simulink model "elevator"  (R2020a)
settings: Solver=VariableStepAuto  StartTime=0.0  StopTime=inf  RelTol=1e-3
PreLoadFcn:
  | slplc.api.loadDataTypes;
undefined symbols (not defined in the file): BOOL, DINT, INT, slplc
libraries: simulink x1
(part 23 of 38)

== system elevator/PLCControllerSuite/__Logic/Task/Program/__Logic/XIO2/BlockEnableRead ==
  __CoreLabelRead : Subsystem  Tag=CoreVarReadBlock  DisableCoverage=on  TreatAsAtomicUnit=on  mask{PLCBlockType=CoreLabelRead}
      mask init:
      | slplc.callbacks.initRoutineLabelRead(gcb);
      mask Help: web([docroot '/plccoder/ref/__corelabelread' '.html']);
      mask DialogControl PLCBlockTitle Prompt: Core Label Read
  Out1 : Outport  VectorParamsAs1DForOutWhenUnconnected=off
  wires:
  __CoreLabelRead/1(Out1) -> Out1/1

== system elevator/PLCControllerSuite/__Logic/Task/Program/__Logic/XIO2/Instruction_Enable ==
  Rung-condition-in : Inport  OutDataTypeStr=BOOL
  Enable : EnablePort
  Logical Operator : Logic  OutDataTypeStr=BOOL
  NOT : Logic  DisableCoverage=on  Operator=NOT  IconShape=distinctive  OutDataTypeStr=BOOL
  __CoreVarRead : Subsystem  Tag=CoreVarReadBlock  DisableCoverage=on  TreatAsAtomicUnit=on  mask{PLCBlockType=CoreVarRead}
      mask init:
      | slplc.callbacks.initCoreVariable(gcb, 'read');
      mask Help: web([docroot '/plccoder/ref/__corevarread' '.html']);
      mask DialogControl PLCBlockTitle Prompt: Core Variable Read
  Rung-condition-out : Outport  VectorParamsAs1DForOutWhenUnconnected=off
  wires:
  NOT/1 -> Logical Operator/2  "~DataBit"
  __CoreVarRead/1(y) -> NOT/1  "DataBit"
  Logical Operator/1 -> Rung-condition-out/1  "Rung-condition-out"
  Rung-condition-in/1 -> Logical Operator/1  "Rung-condition-in"

== system elevator/PLCControllerSuite/__Logic/Task/Program/__Logic/XIO2/RungInOverride ==
  In1 : Inport
  AND : Logic  AllPortsSameDT=off  OutDataTypeStr=boolean
  ForceRungInFalseRead : Subsystem  DisableCoverage=on  TreatAsAtomicUnit=on  mask{PLCLabelTag=_Force_RungIn_False, PLCBlockType=ForceRungInFalseRead}
      mask prompts: PLCLabelTag "Label Tag:"
      mask init:
      | block = gcb;
      | maskObj = Simulink.Mask.get(block);
      | maskObj.Display = sprintf('disp(''%s'');', PLCLabelTag);
      mask Help: web([docroot '/plccoder/ref/forcerunginfalseread' '.html']);
      mask DialogControl PLCBlockTitle Prompt: Force Rung-In False Read
      mask Display: disp('_Force_RungIn_False');
  NOT : Logic  Operator=NOT  IconShape=distinctive  AllPortsSameDT=off  OutDataTypeStr=boolean
  Out1 : Outport  VectorParamsAs1DForOutWhenUnconnected=off
  wires:
  NOT/1 -> AND/1
  ForceRungInFalseRead/1(Out1) -> NOT/1
  In1/1 -> AND/2
  AND/1 -> Out1/1

== system elevator/PLCControllerSuite/__Logic/Task/Program/__Logic/XIO2/__CoreVarRead ==
  DataRead : DataStoreRead  DataStoreName=xxx_PLC_VAR_AtFloor2
  y : Outport  VectorParamsAs1DForOutWhenUnconnected=off
  wires:
  DataRead/1 -> y/1

== system elevator/PLCControllerSuite/__Logic/Task/Program/__Logic/XIO20/BlockEnableRead ==
  __CoreLabelRead : Subsystem  Tag=CoreVarReadBlock  DisableCoverage=on  TreatAsAtomicUnit=on  mask{PLCBlockType=CoreLabelRead}
      mask init:
      | slplc.callbacks.initRoutineLabelRead(gcb);
      mask Help: web([docroot '/plccoder/ref/__corelabelread' '.html']);
      mask DialogControl PLCBlockTitle Prompt: Core Label Read
  Out1 : Outport  VectorParamsAs1DForOutWhenUnconnected=off
  wires:
  __CoreLabelRead/1(Out1) -> Out1/1

== system elevator/PLCControllerSuite/__Logic/Task/Program/__Logic/XIO20/Instruction_Enable ==
  Rung-condition-in : Inport  OutDataTypeStr=BOOL
  Enable : EnablePort
  Logical Operator : Logic  OutDataTypeStr=BOOL
  NOT : Logic  DisableCoverage=on  Operator=NOT  IconShape=distinctive  OutDataTypeStr=BOOL
  __CoreVarRead : Subsystem  Tag=CoreVarReadBlock  DisableCoverage=on  TreatAsAtomicUnit=on  mask{PLCBlockType=CoreVarRead}
      mask init:
      | slplc.callbacks.initCoreVariable(gcb, 'read');
      mask Help: web([docroot '/plccoder/ref/__corevarread' '.html']);
      mask DialogControl PLCBlockTitle Prompt: Core Variable Read
  Rung-condition-out : Outport  VectorParamsAs1DForOutWhenUnconnected=off
  wires:
  NOT/1 -> Logical Operator/2  "~DataBit"
  __CoreVarRead/1(y) -> NOT/1  "DataBit"
  Logical Operator/1 -> Rung-condition-out/1  "Rung-condition-out"
  Rung-condition-in/1 -> Logical Operator/1  "Rung-condition-in"

== system elevator/PLCControllerSuite/__Logic/Task/Program/__Logic/XIO20/RungInOverride ==
  In1 : Inport
  AND : Logic  AllPortsSameDT=off  OutDataTypeStr=boolean
  ForceRungInFalseRead : Subsystem  DisableCoverage=on  TreatAsAtomicUnit=on  mask{PLCLabelTag=_Force_RungIn_False, PLCBlockType=ForceRungInFalseRead}
      mask prompts: PLCLabelTag "Label Tag:"
      mask init:
      | block = gcb;
      | maskObj = Simulink.Mask.get(block);
      | maskObj.Display = sprintf('disp(''%s'');', PLCLabelTag);
      mask Help: web([docroot '/plccoder/ref/forcerunginfalseread' '.html']);
      mask DialogControl PLCBlockTitle Prompt: Force Rung-In False Read
      mask Display: disp('_Force_RungIn_False');
  NOT : Logic  Operator=NOT  IconShape=distinctive  AllPortsSameDT=off  OutDataTypeStr=boolean
  Out1 : Outport  VectorParamsAs1DForOutWhenUnconnected=off
  wires:
  NOT/1 -> AND/1
  ForceRungInFalseRead/1(Out1) -> NOT/1
  In1/1 -> AND/2
  AND/1 -> Out1/1

== system elevator/PLCControllerSuite/__Logic/Task/Program/__Logic/XIO20/__CoreVarRead ==
  DataRead : DataStoreRead  DataStoreName=xxx_PLC_VAR_AtFloor1
  y : Outport  VectorParamsAs1DForOutWhenUnconnected=off
  wires:
  DataRead/1 -> y/1

== system elevator/PLCControllerSuite/__Logic/Task/Program/__Logic/XIO21/BlockEnableRead ==
  __CoreLabelRead : Subsystem  Tag=CoreVarReadBlock  DisableCoverage=on  TreatAsAtomicUnit=on  mask{PLCBlockType=CoreLabelRead}
      mask init:
      | slplc.callbacks.initRoutineLabelRead(gcb);
      mask Help: web([docroot '/plccoder/ref/__corelabelread' '.html']);
      mask DialogControl PLCBlockTitle Prompt: Core Label Read
  Out1 : Outport  VectorParamsAs1DForOutWhenUnconnected=off
  wires:
  __CoreLabelRead/1(Out1) -> Out1/1

== system elevator/PLCControllerSuite/__Logic/Task/Program/__Logic/XIO21/Instruction_Enable ==
  Rung-condition-in : Inport  OutDataTypeStr=BOOL
  Enable : EnablePort
  Logical Operator : Logic  OutDataTypeStr=BOOL
  NOT : Logic  DisableCoverage=on  Operator=NOT  IconShape=distinctive  OutDataTypeStr=BOOL
  __CoreVarRead : Subsystem  Tag=CoreVarReadBlock  DisableCoverage=on  TreatAsAtomicUnit=on  mask{PLCBlockType=CoreVarRead}
      mask init:
      | slplc.callbacks.initCoreVariable(gcb, 'read');
      mask Help: web([docroot '/plccoder/ref/__corevarread' '.html']);
      mask DialogControl PLCBlockTitle Prompt: Core Variable Read
  Rung-condition-out : Outport  VectorParamsAs1DForOutWhenUnconnected=off
  wires:
  NOT/1 -> Logical Operator/2  "~DataBit"
  __CoreVarRead/1(y) -> NOT/1  "DataBit"
  Logical Operator/1 -> Rung-condition-out/1  "Rung-condition-out"
  Rung-condition-in/1 -> Logical Operator/1  "Rung-condition-in"

== system elevator/PLCControllerSuite/__Logic/Task/Program/__Logic/XIO21/RungInOverride ==
  In1 : Inport
  AND : Logic  AllPortsSameDT=off  OutDataTypeStr=boolean
  ForceRungInFalseRead : Subsystem  DisableCoverage=on  TreatAsAtomicUnit=on  mask{PLCLabelTag=_Force_RungIn_False, PLCBlockType=ForceRungInFalseRead}
      mask prompts: PLCLabelTag "Label Tag:"
      mask init:
      | block = gcb;
      | maskObj = Simulink.Mask.get(block);
      | maskObj.Display = sprintf('disp(''%s'');', PLCLabelTag);
      mask Help: web([docroot '/plccoder/ref/forcerunginfalseread' '.html']);
      mask DialogControl PLCBlockTitle Prompt: Force Rung-In False Read
      mask Display: disp('_Force_RungIn_False');
  NOT : Logic  Operator=NOT  IconShape=distinctive  AllPortsSameDT=off  OutDataTypeStr=boolean
  Out1 : Outport  VectorParamsAs1DForOutWhenUnconnected=off
  wires:
  NOT/1 -> AND/1
  ForceRungInFalseRead/1(Out1) -> NOT/1
  In1/1 -> AND/2
  AND/1 -> Out1/1

== system elevator/PLCControllerSuite/__Logic/Task/Program/__Logic/XIO21/__CoreVarRead ==
  DataRead : DataStoreRead  DataStoreName=xxx_PLC_VAR_AtFloor3
  y : Outport  VectorParamsAs1DForOutWhenUnconnected=off
  wires:
  DataRead/1 -> y/1

== system elevator/PLCControllerSuite/__Logic/Task/Program/__Logic/XIO22/BlockEnableRead ==
  __CoreLabelRead : Subsystem  Tag=CoreVarReadBlock  DisableCoverage=on  TreatAsAtomicUnit=on  mask{PLCBlockType=CoreLabelRead}
      mask init:
      | slplc.callbacks.initRoutineLabelRead(gcb);
      mask Help: web([docroot '/plccoder/ref/__corelabelread' '.html']);
      mask DialogControl PLCBlockTitle Prompt: Core Label Read
  Out1 : Outport  VectorParamsAs1DForOutWhenUnconnected=off
  wires:
  __CoreLabelRead/1(Out1) -> Out1/1

== system elevator/PLCControllerSuite/__Logic/Task/Program/__Logic/XIO22/Instruction_Enable ==
  Rung-condition-in : Inport  OutDataTypeStr=BOOL
  Enable : EnablePort
  Logical Operator : Logic  OutDataTypeStr=BOOL
  NOT : Logic  DisableCoverage=on  Operator=NOT  IconShape=distinctive  OutDataTypeStr=BOOL
  __CoreVarRead : Subsystem  Tag=CoreVarReadBlock  DisableCoverage=on  TreatAsAtomicUnit=on  mask{PLCBlockType=CoreVarRead}
      mask init:
      | slplc.callbacks.initCoreVariable(gcb, 'read');
      mask Help: web([docroot '/plccoder/ref/__corevarread' '.html']);
      mask DialogControl PLCBlockTitle Prompt: Core Variable Read
  Rung-condition-out : Outport  VectorParamsAs1DForOutWhenUnconnected=off
  wires:
  Rung-condition-in/1 -> Logical Operator/1  "Rung-condition-in"
  Logical Operator/1 -> Rung-condition-out/1  "Rung-condition-out"
  __CoreVarRead/1(y) -> NOT/1  "DataBit"
  NOT/1 -> Logical Operator/2  "~DataBit"

== system elevator/PLCControllerSuite/__Logic/Task/Program/__Logic/XIO22/RungInOverride ==
  In1 : Inport
  AND : Logic  AllPortsSameDT=off  OutDataTypeStr=boolean
  ForceRungInFalseRead : Subsystem  DisableCoverage=on  TreatAsAtomicUnit=on  mask{PLCLabelTag=_Force_RungIn_False, PLCBlockType=ForceRungInFalseRead}
      mask prompts: PLCLabelTag "Label Tag:"
      mask init:
      | block = gcb;
      | maskObj = Simulink.Mask.get(block);
      | maskObj.Display = sprintf('disp(''%s'');', PLCLabelTag);
      mask Help: web([docroot '/plccoder/ref/forcerunginfalseread' '.html']);
      mask DialogControl PLCBlockTitle Prompt: Force Rung-In False Read
      mask Display: disp('_Force_RungIn_False');
  NOT : Logic  Operator=NOT  IconShape=distinctive  AllPortsSameDT=off  OutDataTypeStr=boolean
  Out1 : Outport  VectorParamsAs1DForOutWhenUnconnected=off
  wires:
  AND/1 -> Out1/1
  In1/1 -> AND/2
  ForceRungInFalseRead/1(Out1) -> NOT/1
  NOT/1 -> AND/1

== system elevator/PLCControllerSuite/__Logic/Task/Program/__Logic/XIO22/__CoreVarRead ==
  DataRead : DataStoreRead  DataStoreName=xxx_PLC_VAR_AtFloor1
  y : Outport  VectorParamsAs1DForOutWhenUnconnected=off
  wires:
  DataRead/1 -> y/1

== system elevator/PLCControllerSuite/__Logic/Task/Program/__Logic/XIO23/BlockEnableRead ==
  __CoreLabelRead : Subsystem  Tag=CoreVarReadBlock  DisableCoverage=on  TreatAsAtomicUnit=on  mask{PLCBlockType=CoreLabelRead}
      mask init:
      | slplc.callbacks.initRoutineLabelRead(gcb);
      mask Help: web([docroot '/plccoder/ref/__corelabelread' '.html']);
      mask DialogControl PLCBlockTitle Prompt: Core Label Read
  Out1 : Outport  VectorParamsAs1DForOutWhenUnconnected=off
  wires:
  __CoreLabelRead/1(Out1) -> Out1/1

== system elevator/PLCControllerSuite/__Logic/Task/Program/__Logic/XIO23/Instruction_Enable ==
  Rung-condition-in : Inport  OutDataTypeStr=BOOL
  Enable : EnablePort
  Logical Operator : Logic  OutDataTypeStr=BOOL
  NOT : Logic  DisableCoverage=on  Operator=NOT  IconShape=distinctive  OutDataTypeStr=BOOL
  __CoreVarRead : Subsystem  Tag=CoreVarReadBlock  DisableCoverage=on  TreatAsAtomicUnit=on  mask{PLCBlockType=CoreVarRead}
      mask init:
      | slplc.callbacks.initCoreVariable(gcb, 'read');
      mask Help: web([docroot '/plccoder/ref/__corevarread' '.html']);
      mask DialogControl PLCBlockTitle Prompt: Core Variable Read
  Rung-condition-out : Outport  VectorParamsAs1DForOutWhenUnconnected=off
  wires:
  Rung-condition-in/1 -> Logical Operator/1  "Rung-condition-in"
  Logical Operator/1 -> Rung-condition-out/1  "Rung-condition-out"
  __CoreVarRead/1(y) -> NOT/1  "DataBit"
  NOT/1 -> Logical Operator/2  "~DataBit"

== system elevator/PLCControllerSuite/__Logic/Task/Program/__Logic/XIO23/RungInOverride ==
  In1 : Inport
  AND : Logic  AllPortsSameDT=off  OutDataTypeStr=boolean
  ForceRungInFalseRead : Subsystem  DisableCoverage=on  TreatAsAtomicUnit=on  mask{PLCLabelTag=_Force_RungIn_False, PLCBlockType=ForceRungInFalseRead}
      mask prompts: PLCLabelTag "Label Tag:"
      mask init:
      | block = gcb;
      | maskObj = Simulink.Mask.get(block);
      | maskObj.Display = sprintf('disp(''%s'');', PLCLabelTag);
      mask Help: web([docroot '/plccoder/ref/forcerunginfalseread' '.html']);
      mask DialogControl PLCBlockTitle Prompt: Force Rung-In False Read
      mask Display: disp('_Force_RungIn_False');
  NOT : Logic  Operator=NOT  IconShape=distinctive  AllPortsSameDT=off  OutDataTypeStr=boolean
  Out1 : Outport  VectorParamsAs1DForOutWhenUnconnected=off
  wires:
  AND/1 -> Out1/1
  In1/1 -> AND/2
  ForceRungInFalseRead/1(Out1) -> NOT/1
  NOT/1 -> AND/1

== system elevator/PLCControllerSuite/__Logic/Task/Program/__Logic/XIO23/__CoreVarRead ==
  DataRead : DataStoreRead  DataStoreName=xxx_PLC_VAR_AtFloor1
  y : Outport  VectorParamsAs1DForOutWhenUnconnected=off
  wires:
  DataRead/1 -> y/1

== system elevator/PLCControllerSuite/__Logic/Task/Program/__Logic/XIO24/BlockEnableRead ==
  __CoreLabelRead : Subsystem  Tag=CoreVarReadBlock  DisableCoverage=on  TreatAsAtomicUnit=on  mask{PLCBlockType=CoreLabelRead}
      mask init:
      | slplc.callbacks.initRoutineLabelRead(gcb);
      mask Help: web([docroot '/plccoder/ref/__corelabelread' '.html']);
      mask DialogControl PLCBlockTitle Prompt: Core Label Read
  Out1 : Outport  VectorParamsAs1DForOutWhenUnconnected=off
  wires:
  __CoreLabelRead/1(Out1) -> Out1/1

== system elevator/PLCControllerSuite/__Logic/Task/Program/__Logic/XIO24/Instruction_Enable ==
  Rung-condition-in : Inport  OutDataTypeStr=BOOL
  Enable : EnablePort
  Logical Operator : Logic  OutDataTypeStr=BOOL
  NOT : Logic  DisableCoverage=on  Operator=NOT  IconShape=distinctive  OutDataTypeStr=BOOL
  __CoreVarRead : Subsystem  Tag=CoreVarReadBlock  DisableCoverage=on  TreatAsAtomicUnit=on  mask{PLCBlockType=CoreVarRead}
      mask init:
      | slplc.callbacks.initCoreVariable(gcb, 'read');
      mask Help: web([docroot '/plccoder/ref/__corevarread' '.html']);
      mask DialogControl PLCBlockTitle Prompt: Core Variable Read
  Rung-condition-out : Outport  VectorParamsAs1DForOutWhenUnconnected=off
  wires:
  NOT/1 -> Logical Operator/2  "~DataBit"
  __CoreVarRead/1(y) -> NOT/1  "DataBit"
  Logical Operator/1 -> Rung-condition-out/1  "Rung-condition-out"
  Rung-condition-in/1 -> Logical Operator/1  "Rung-condition-in"

== system elevator/PLCControllerSuite/__Logic/Task/Program/__Logic/XIO24/RungInOverride ==
  In1 : Inport
  AND : Logic  AllPortsSameDT=off  OutDataTypeStr=boolean
  ForceRungInFalseRead : Subsystem  DisableCoverage=on  TreatAsAtomicUnit=on  mask{PLCLabelTag=_Force_RungIn_False, PLCBlockType=ForceRungInFalseRead}
      mask prompts: PLCLabelTag "Label Tag:"
      mask init:
      | block = gcb;
      | maskObj = Simulink.Mask.get(block);
      | maskObj.Display = sprintf('disp(''%s'');', PLCLabelTag);
      mask Help: web([docroot '/plccoder/ref/forcerunginfalseread' '.html']);
      mask DialogControl PLCBlockTitle Prompt: Force Rung-In False Read
      mask Display: disp('_Force_RungIn_False');
  NOT : Logic  Operator=NOT  IconShape=distinctive  AllPortsSameDT=off  OutDataTypeStr=boolean
  Out1 : Outport  VectorParamsAs1DForOutWhenUnconnected=off
  wires:
  NOT/1 -> AND/1
  ForceRungInFalseRead/1(Out1) -> NOT/1
  In1/1 -> AND/2
  AND/1 -> Out1/1

== system elevator/PLCControllerSuite/__Logic/Task/Program/__Logic/XIO24/__CoreVarRead ==
  DataRead : DataStoreRead  DataStoreName=xxx_PLC_VAR_AtFloor2
  y : Outport  VectorParamsAs1DForOutWhenUnconnected=off
  wires:
  DataRead/1 -> y/1

== system elevator/PLCControllerSuite/__Logic/Task/Program/__Logic/XIO25/BlockEnableRead ==
  __CoreLabelRead : Subsystem  Tag=CoreVarReadBlock  DisableCoverage=on  TreatAsAtomicUnit=on  mask{PLCBlockType=CoreLabelRead}
      mask init:
      | slplc.callbacks.initRoutineLabelRead(gcb);
      mask Help: web([docroot '/plccoder/ref/__corelabelread' '.html']);
      mask DialogControl PLCBlockTitle Prompt: Core Label Read
  Out1 : Outport  VectorParamsAs1DForOutWhenUnconnected=off
  wires:
  __CoreLabelRead/1(Out1) -> Out1/1

== system elevator/PLCControllerSuite/__Logic/Task/Program/__Logic/XIO25/Instruction_Enable ==
  Rung-condition-in : Inport  OutDataTypeStr=BOOL
  Enable : EnablePort
  Logical Operator : Logic  OutDataTypeStr=BOOL
  NOT : Logic  DisableCoverage=on  Operator=NOT  IconShape=distinctive  OutDataTypeStr=BOOL
  __CoreVarRead : Subsystem  Tag=CoreVarReadBlock  DisableCoverage=on  TreatAsAtomicUnit=on  mask{PLCBlockType=CoreVarRead}
      mask init:
      | slplc.callbacks.initCoreVariable(gcb, 'read');
      mask Help: web([docroot '/plccoder/ref/__corevarread' '.html']);
      mask DialogControl PLCBlockTitle Prompt: Core Variable Read
  Rung-condition-out : Outport  VectorParamsAs1DForOutWhenUnconnected=off
  wires:
  NOT/1 -> Logical Operator/2  "~DataBit"
  __CoreVarRead/1(y) -> NOT/1  "DataBit"
  Logical Operator/1 -> Rung-condition-out/1  "Rung-condition-out"
  Rung-condition-in/1 -> Logical Operator/1  "Rung-condition-in"

== system elevator/PLCControllerSuite/__Logic/Task/Program/__Logic/XIO25/RungInOverride ==
  In1 : Inport
  AND : Logic  AllPortsSameDT=off  OutDataTypeStr=boolean
  ForceRungInFalseRead : Subsystem  DisableCoverage=on  TreatAsAtomicUnit=on  mask{PLCLabelTag=_Force_RungIn_False, PLCBlockType=ForceRungInFalseRead}
      mask prompts: PLCLabelTag "Label Tag:"
      mask init:
      | block = gcb;
      | maskObj = Simulink.Mask.get(block);
      | maskObj.Display = sprintf('disp(''%s'');', PLCLabelTag);
      mask Help: web([docroot '/plccoder/ref/forcerunginfalseread' '.html']);
      mask DialogControl PLCBlockTitle Prompt: Force Rung-In False Read
      mask Display: disp('_Force_RungIn_False');
  NOT : Logic  Operator=NOT  IconShape=distinctive  AllPortsSameDT=off  OutDataTypeStr=boolean
  Out1 : Outport  VectorParamsAs1DForOutWhenUnconnected=off
  wires:
  NOT/1 -> AND/1
  ForceRungInFalseRead/1(Out1) -> NOT/1
  In1/1 -> AND/2
  AND/1 -> Out1/1

== system elevator/PLCControllerSuite/__Logic/Task/Program/__Logic/XIO25/__CoreVarRead ==
  DataRead : DataStoreRead  DataStoreName=xxx_PLC_VAR_LSTDIRUP
  y : Outport  VectorParamsAs1DForOutWhenUnconnected=off
  wires:
  DataRead/1 -> y/1

== system elevator/PLCControllerSuite/__Logic/Task/Program/__Logic/XIO26/BlockEnableRead ==
  __CoreLabelRead : Subsystem  Tag=CoreVarReadBlock  DisableCoverage=on  TreatAsAtomicUnit=on  mask{PLCBlockType=CoreLabelRead}
      mask init:
      | slplc.callbacks.initRoutineLabelRead(gcb);
      mask Help: web([docroot '/plccoder/ref/__corelabelread' '.html']);
      mask DialogControl PLCBlockTitle Prompt: Core Label Read
  Out1 : Outport  VectorParamsAs1DForOutWhenUnconnected=off
  wires:
  __CoreLabelRead/1(Out1) -> Out1/1

== system elevator/PLCControllerSuite/__Logic/Task/Program/__Logic/XIO26/Instruction_Enable ==
  Rung-condition-in : Inport  OutDataTypeStr=BOOL
  Enable : EnablePort
  Logical Operator : Logic  OutDataTypeStr=BOOL
  NOT : Logic  DisableCoverage=on  Operator=NOT  IconShape=distinctive  OutDataTypeStr=BOOL
  __CoreVarRead : Subsystem  Tag=CoreVarReadBlock  DisableCoverage=on  TreatAsAtomicUnit=on  mask{PLCBlockType=CoreVarRead}
      mask init:
      | slplc.callbacks.initCoreVariable(gcb, 'read');
      mask Help: web([docroot '/plccoder/ref/__corevarread' '.html']);
      mask DialogControl PLCBlockTitle Prompt: Core Variable Read
  Rung-condition-out : Outport  VectorParamsAs1DForOutWhenUnconnected=off
  wires:
  Rung-condition-in/1 -> Logical Operator/1  "Rung-condition-in"
  Logical Operator/1 -> Rung-condition-out/1  "Rung-condition-out"
  __CoreVarRead/1(y) -> NOT/1  "DataBit"
  NOT/1 -> Logical Operator/2  "~DataBit"

== system elevator/PLCControllerSuite/__Logic/Task/Program/__Logic/XIO26/RungInOverride ==
  In1 : Inport
  AND : Logic  AllPortsSameDT=off  OutDataTypeStr=boolean
  ForceRungInFalseRead : Subsystem  DisableCoverage=on  TreatAsAtomicUnit=on  mask{PLCLabelTag=_Force_RungIn_False, PLCBlockType=ForceRungInFalseRead}
      mask prompts: PLCLabelTag "Label Tag:"
      mask init:
      | block = gcb;
      | maskObj = Simulink.Mask.get(block);
      | maskObj.Display = sprintf('disp(''%s'');', PLCLabelTag);
      mask Help: web([docroot '/plccoder/ref/forcerunginfalseread' '.html']);
      mask DialogControl PLCBlockTitle Prompt: Force Rung-In False Read
      mask Display: disp('_Force_RungIn_False');
  NOT : Logic  Operator=NOT  IconShape=distinctive  AllPortsSameDT=off  OutDataTypeStr=boolean
  Out1 : Outport  VectorParamsAs1DForOutWhenUnconnected=off
  wires:
  AND/1 -> Out1/1
  In1/1 -> AND/2
  ForceRungInFalseRead/1(Out1) -> NOT/1
  NOT/1 -> AND/1

== system elevator/PLCControllerSuite/__Logic/Task/Program/__Logic/XIO26/__CoreVarRead ==
  DataRead : DataStoreRead  DataStoreName=xxx_PLC_VAR_MemoryGoUp
  y : Outport  VectorParamsAs1DForOutWhenUnconnected=off
  wires:
  DataRead/1 -> y/1

== system elevator/PLCControllerSuite/__Logic/Task/Program/__Logic/XIO27/BlockEnableRead ==
  __CoreLabelRead : Subsystem  Tag=CoreVarReadBlock  DisableCoverage=on  TreatAsAtomicUnit=on  mask{PLCBlockType=CoreLabelRead}
      mask init:
      | slplc.callbacks.initRoutineLabelRead(gcb);
      mask Help: web([docroot '/plccoder/ref/__corelabelread' '.html']);
      mask DialogControl PLCBlockTitle Prompt: Core Label Read
  Out1 : Outport  VectorParamsAs1DForOutWhenUnconnected=off
  wires:
  __CoreLabelRead/1(Out1) -> Out1/1

== system elevator/PLCControllerSuite/__Logic/Task/Program/__Logic/XIO27/Instruction_Enable ==
  Rung-condition-in : Inport  OutDataTypeStr=BOOL
  Enable : EnablePort
  Logical Operator : Logic  OutDataTypeStr=BOOL
  NOT : Logic  DisableCoverage=on  Operator=NOT  IconShape=distinctive  OutDataTypeStr=BOOL
  __CoreVarRead : Subsystem  Tag=CoreVarReadBlock  DisableCoverage=on  TreatAsAtomicUnit=on  mask{PLCBlockType=CoreVarRead}
      mask init:
      | slplc.callbacks.initCoreVariable(gcb, 'read');
      mask Help: web([docroot '/plccoder/ref/__corevarread' '.html']);
      mask DialogControl PLCBlockTitle Prompt: Core Variable Read
  Rung-condition-out : Outport  VectorParamsAs1DForOutWhenUnconnected=off
  wires:
  Rung-condition-in/1 -> Logical Operator/1  "Rung-condition-in"
  Logical Operator/1 -> Rung-condition-out/1  "Rung-condition-out"
  __CoreVarRead/1(y) -> NOT/1  "DataBit"
  NOT/1 -> Logical Operator/2  "~DataBit"

== system elevator/PLCControllerSuite/__Logic/Task/Program/__Logic/XIO27/RungInOverride ==
  In1 : Inport
  AND : Logic  AllPortsSameDT=off  OutDataTypeStr=boolean
  ForceRungInFalseRead : Subsystem  DisableCoverage=on  TreatAsAtomicUnit=on  mask{PLCLabelTag=_Force_RungIn_False, PLCBlockType=ForceRungInFalseRead}
      mask prompts: PLCLabelTag "Label Tag:"
      mask init:
      | block = gcb;
      | maskObj = Simulink.Mask.get(block);
      | maskObj.Display = sprintf('disp(''%s'');', PLCLabelTag);
      mask Help: web([docroot '/plccoder/ref/forcerunginfalseread' '.html']);
      mask DialogControl PLCBlockTitle Prompt: Force Rung-In False Read
      mask Display: disp('_Force_RungIn_False');
  NOT : Logic  Operator=NOT  IconShape=distinctive  AllPortsSameDT=off  OutDataTypeStr=boolean
  Out1 : Outport  VectorParamsAs1DForOutWhenUnconnected=off
  wires:
  AND/1 -> Out1/1
  In1/1 -> AND/2
  ForceRungInFalseRead/1(Out1) -> NOT/1
  NOT/1 -> AND/1

== system elevator/PLCControllerSuite/__Logic/Task/Program/__Logic/XIO27/__CoreVarRead ==
  DataRead : DataStoreRead  DataStoreName=xxx_PLC_VAR_GOINGDN
  y : Outport  VectorParamsAs1DForOutWhenUnconnected=off
  wires:
  DataRead/1 -> y/1

== system elevator/PLCControllerSuite/__Logic/Task/Program/__Logic/XIO28/BlockEnableRead ==
  __CoreLabelRead : Subsystem  Tag=CoreVarReadBlock  DisableCoverage=on  TreatAsAtomicUnit=on  mask{PLCBlockType=CoreLabelRead}
      mask init:
      | slplc.callbacks.initRoutineLabelRead(gcb);
      mask Help: web([docroot '/plccoder/ref/__corelabelread' '.html']);
      mask DialogControl PLCBlockTitle Prompt: Core Label Read
  Out1 : Outport  VectorParamsAs1DForOutWhenUnconnected=off
  wires:
  __CoreLabelRead/1(Out1) -> Out1/1

== system elevator/PLCControllerSuite/__Logic/Task/Program/__Logic/XIO28/Instruction_Enable ==
  Rung-condition-in : Inport  OutDataTypeStr=BOOL
  Enable : EnablePort
  Logical Operator : Logic  OutDataTypeStr=BOOL
  NOT : Logic  DisableCoverage=on  Operator=NOT  IconShape=distinctive  OutDataTypeStr=BOOL
  __CoreVarRead : Subsystem  Tag=CoreVarReadBlock  DisableCoverage=on  TreatAsAtomicUnit=on  mask{PLCBlockType=CoreVarRead}
      mask init:
      | slplc.callbacks.initCoreVariable(gcb, 'read');
      mask Help: web([docroot '/plccoder/ref/__corevarread' '.html']);
      mask DialogControl PLCBlockTitle Prompt: Core Variable Read
  Rung-condition-out : Outport  VectorParamsAs1DForOutWhenUnconnected=off
  wires:
  NOT/1 -> Logical Operator/2  "~DataBit"
  __CoreVarRead/1(y) -> NOT/1  "DataBit"
  Logical Operator/1 -> Rung-condition-out/1  "Rung-condition-out"
  Rung-condition-in/1 -> Logical Operator/1  "Rung-condition-in"

== system elevator/PLCControllerSuite/__Logic/Task/Program/__Logic/XIO28/RungInOverride ==
  In1 : Inport
  AND : Logic  AllPortsSameDT=off  OutDataTypeStr=boolean
  ForceRungInFalseRead : Subsystem  DisableCoverage=on  TreatAsAtomicUnit=on  mask{PLCLabelTag=_Force_RungIn_False, PLCBlockType=ForceRungInFalseRead}
      mask prompts: PLCLabelTag "Label Tag:"
      mask init:
      | block = gcb;
      | maskObj = Simulink.Mask.get(block);
      | maskObj.Display = sprintf('disp(''%s'');', PLCLabelTag);
      mask Help: web([docroot '/plccoder/ref/forcerunginfalseread' '.html']);
      mask DialogControl PLCBlockTitle Prompt: Force Rung-In False Read
      mask Display: disp('_Force_RungIn_False');
  NOT : Logic  Operator=NOT  IconShape=distinctive  AllPortsSameDT=off  OutDataTypeStr=boolean
  Out1 : Outport  VectorParamsAs1DForOutWhenUnconnected=off
  wires:
  NOT/1 -> AND/1
  ForceRungInFalseRead/1(Out1) -> NOT/1
  In1/1 -> AND/2
  AND/1 -> Out1/1

== system elevator/PLCControllerSuite/__Logic/Task/Program/__Logic/XIO28/__CoreVarRead ==
  DataRead : DataStoreRead  DataStoreName=xxx_PLC_VAR_RMPDNKIL
  y : Outport  VectorParamsAs1DForOutWhenUnconnected=off
  wires:
  DataRead/1 -> y/1

== system elevator/PLCControllerSuite/__Logic/Task/Program/__Logic/XIO29/BlockEnableRead ==
  __CoreLabelRead : Subsystem  Tag=CoreVarReadBlock  DisableCoverage=on  TreatAsAtomicUnit=on  mask{PLCBlockType=CoreLabelRead}
      mask init:
      | slplc.callbacks.initRoutineLabelRead(gcb);
      mask Help: web([docroot '/plccoder/ref/__corelabelread' '.html']);
      mask DialogControl PLCBlockTitle Prompt: Core Label Read
  Out1 : Outport  VectorParamsAs1DForOutWhenUnconnected=off
  wires:
  __CoreLabelRead/1(Out1) -> Out1/1

== system elevator/PLCControllerSuite/__Logic/Task/Program/__Logic/XIO29/Instruction_Enable ==
  Rung-condition-in : Inport  OutDataTypeStr=BOOL
  Enable : EnablePort
  Logical Operator : Logic  OutDataTypeStr=BOOL
  NOT : Logic  DisableCoverage=on  Operator=NOT  IconShape=distinctive  OutDataTypeStr=BOOL
  __CoreVarRead : Subsystem  Tag=CoreVarReadBlock  DisableCoverage=on  TreatAsAtomicUnit=on  mask{PLCBlockType=CoreVarRead}
      mask init:
      | slplc.callbacks.initCoreVariable(gcb, 'read');
      mask Help: web([docroot '/plccoder/ref/__corevarread' '.html']);
      mask DialogControl PLCBlockTitle Prompt: Core Variable Read
  Rung-condition-out : Outport  VectorParamsAs1DForOutWhenUnconnected=off
  wires:
  NOT/1 -> Logical Operator/2  "~DataBit"
  __CoreVarRead/1(y) -> NOT/1  "DataBit"
  Logical Operator/1 -> Rung-condition-out/1  "Rung-condition-out"
  Rung-condition-in/1 -> Logical Operator/1  "Rung-condition-in"

== system elevator/PLCControllerSuite/__Logic/Task/Program/__Logic/XIO29/RungInOverride ==
  In1 : Inport
  AND : Logic  AllPortsSameDT=off  OutDataTypeStr=boolean
  ForceRungInFalseRead : Subsystem  DisableCoverage=on  TreatAsAtomicUnit=on  mask{PLCLabelTag=_Force_RungIn_False, PLCBlockType=ForceRungInFalseRead}
      mask prompts: PLCLabelTag "Label Tag:"
      mask init:
      | block = gcb;
      | maskObj = Simulink.Mask.get(block);
      | maskObj.Display = sprintf('disp(''%s'');', PLCLabelTag);
      mask Help: web([docroot '/plccoder/ref/forcerunginfalseread' '.html']);
      mask DialogControl PLCBlockTitle Prompt: Force Rung-In False Read
      mask Display: disp('_Force_RungIn_False');
  NOT : Logic  Operator=NOT  IconShape=distinctive  AllPortsSameDT=off  OutDataTypeStr=boolean
  Out1 : Outport  VectorParamsAs1DForOutWhenUnconnected=off
  wires:
  NOT/1 -> AND/1
  ForceRungInFalseRead/1(Out1) -> NOT/1
  In1/1 -> AND/2
  AND/1 -> Out1/1

== system elevator/PLCControllerSuite/__Logic/Task/Program/__Logic/XIO29/__CoreVarRead ==
  DataRead : DataStoreRead  DataStoreName=xxx_PLC_VAR_AtFloor2
  y : Outport  VectorParamsAs1DForOutWhenUnconnected=off
  wires:
  DataRead/1 -> y/1

== system elevator/PLCControllerSuite/__Logic/Task/Program/__Logic/XIO3/BlockEnableRead ==
  __CoreLabelRead : Subsystem  Tag=CoreVarReadBlock  DisableCoverage=on  TreatAsAtomicUnit=on  mask{PLCBlockType=CoreLabelRead}
      mask init:
      | slplc.callbacks.initRoutineLabelRead(gcb);
      mask Help: web([docroot '/plccoder/ref/__corelabelread' '.html']);
      mask DialogControl PLCBlockTitle Prompt: Core Label Read
  Out1 : Outport  VectorParamsAs1DForOutWhenUnconnected=off
  wires:
  __CoreLabelRead/1(Out1) -> Out1/1

== system elevator/PLCControllerSuite/__Logic/Task/Program/__Logic/XIO3/Instruction_Enable ==
  Rung-condition-in : Inport  OutDataTypeStr=BOOL
  Enable : EnablePort
  Logical Operator : Logic  OutDataTypeStr=BOOL
  NOT : Logic  DisableCoverage=on  Operator=NOT  IconShape=distinctive  OutDataTypeStr=BOOL
  __CoreVarRead : Subsystem  Tag=CoreVarReadBlock  DisableCoverage=on  TreatAsAtomicUnit=on  mask{PLCBlockType=CoreVarRead}
      mask init:
      | slplc.callbacks.initCoreVariable(gcb, 'read');
      mask Help: web([docroot '/plccoder/ref/__corevarread' '.html']);
      mask DialogControl PLCBlockTitle Prompt: Core Variable Read
  Rung-condition-out : Outport  VectorParamsAs1DForOutWhenUnconnected=off
  wires:
  Rung-condition-in/1 -> Logical Operator/1  "Rung-condition-in"
  Logical Operator/1 -> Rung-condition-out/1  "Rung-condition-out"
  __CoreVarRead/1(y) -> NOT/1  "DataBit"
  NOT/1 -> Logical Operator/2  "~DataBit"

== system elevator/PLCControllerSuite/__Logic/Task/Program/__Logic/XIO3/RungInOverride ==
  In1 : Inport
  AND : Logic  AllPortsSameDT=off  OutDataTypeStr=boolean
  ForceRungInFalseRead : Subsystem  DisableCoverage=on  TreatAsAtomicUnit=on  mask{PLCLabelTag=_Force_RungIn_False, PLCBlockType=ForceRungInFalseRead}
      mask prompts: PLCLabelTag "Label Tag:"
      mask init:
      | block = gcb;
      | maskObj = Simulink.Mask.get(block);
      | maskObj.Display = sprintf('disp(''%s'');', PLCLabelTag);
      mask Help: web([docroot '/plccoder/ref/forcerunginfalseread' '.html']);
      mask DialogControl PLCBlockTitle Prompt: Force Rung-In False Read
      mask Display: disp('_Force_RungIn_False');
  NOT : Logic  Operator=NOT  IconShape=distinctive  AllPortsSameDT=off  OutDataTypeStr=boolean
  Out1 : Outport  VectorParamsAs1DForOutWhenUnconnected=off
  wires:
  AND/1 -> Out1/1
  In1/1 -> AND/2
  ForceRungInFalseRead/1(Out1) -> NOT/1
  NOT/1 -> AND/1

== system elevator/PLCControllerSuite/__Logic/Task/Program/__Logic/XIO3/__CoreVarRead ==
  DataRead : DataStoreRead  DataStoreName=xxx_PLC_VAR_AtFloor3
  y : Outport  VectorParamsAs1DForOutWhenUnconnected=off
  wires:
  DataRead/1 -> y/1

== system elevator/PLCControllerSuite/__Logic/Task/Program/__Logic/XIO30/BlockEnableRead ==
  __CoreLabelRead : Subsystem  Tag=CoreVarReadBlock  DisableCoverage=on  TreatAsAtomicUnit=on  mask{PLCBlockType=CoreLabelRead}
      mask init:
      | slplc.callbacks.initRoutineLabelRead(gcb);
      mask Help: web([docroot '/plccoder/ref/__corelabelread' '.html']);
      mask DialogControl PLCBlockTitle Prompt: Core Label Read
  Out1 : Outport  VectorParamsAs1DForOutWhenUnconnected=off
  wires:
  __CoreLabelRead/1(Out1) -> Out1/1

== system elevator/PLCControllerSuite/__Logic/Task/Program/__Logic/XIO30/Instruction_Enable ==
  Rung-condition-in : Inport  OutDataTypeStr=BOOL
  Enable : EnablePort
  Logical Operator : Logic  OutDataTypeStr=BOOL
  NOT : Logic  DisableCoverage=on  Operator=NOT  IconShape=distinctive  OutDataTypeStr=BOOL
  __CoreVarRead : Subsystem  Tag=CoreVarReadBlock  DisableCoverage=on  TreatAsAtomicUnit=on  mask{PLCBlockType=CoreVarRead}
      mask init:
      | slplc.callbacks.initCoreVariable(gcb, 'read');
      mask Help: web([docroot '/plccoder/ref/__corevarread' '.html']);
      mask DialogControl PLCBlockTitle Prompt: Core Variable Read
  Rung-condition-out : Outport  VectorParamsAs1DForOutWhenUnconnected=off
  wires:
  Rung-condition-in/1 -> Logical Operator/1  "Rung-condition-in"
  Logical Operator/1 -> Rung-condition-out/1  "Rung-condition-out"
  __CoreVarRead/1(y) -> NOT/1  "DataBit"
  NOT/1 -> Logical Operator/2  "~DataBit"

== system elevator/PLCControllerSuite/__Logic/Task/Program/__Logic/XIO30/RungInOverride ==
  In1 : Inport
  AND : Logic  AllPortsSameDT=off  OutDataTypeStr=boolean
  ForceRungInFalseRead : Subsystem  DisableCoverage=on  TreatAsAtomicUnit=on  mask{PLCLabelTag=_Force_RungIn_False, PLCBlockType=ForceRungInFalseRead}
      mask prompts: PLCLabelTag "Label Tag:"
      mask init:
      | block = gcb;
      | maskObj = Simulink.Mask.get(block);
      | maskObj.Display = sprintf('disp(''%s'');', PLCLabelTag);
      mask Help: web([docroot '/plccoder/ref/forcerunginfalseread' '.html']);
      mask DialogControl PLCBlockTitle Prompt: Force Rung-In False Read
      mask Display: disp('_Force_RungIn_False');
  NOT : Logic  Operator=NOT  IconShape=distinctive  AllPortsSameDT=off  OutDataTypeStr=boolean
  Out1 : Outport  VectorParamsAs1DForOutWhenUnconnected=off
  wires:
  AND/1 -> Out1/1
  In1/1 -> AND/2
  ForceRungInFalseRead/1(Out1) -> NOT/1
  NOT/1 -> AND/1

== system elevator/PLCControllerSuite/__Logic/Task/Program/__Logic/XIO30/__CoreVarRead ==
  DataRead : DataStoreRead  DataStoreName=xxx_PLC_VAR_RMPUPKIL
  y : Outport  VectorParamsAs1DForOutWhenUnconnected=off
  wires:
  DataRead/1 -> y/1

== system elevator/PLCControllerSuite/__Logic/Task/Program/__Logic/XIO31/BlockEnableRead ==
  __CoreLabelRead : Subsystem  Tag=CoreVarReadBlock  DisableCoverage=on  TreatAsAtomicUnit=on  mask{PLCBlockType=CoreLabelRead}
      mask init:
      | slplc.callbacks.initRoutineLabelRead(gcb);
      mask Help: web([docroot '/plccoder/ref/__corelabelread' '.html']);
      mask DialogControl PLCBlockTitle Prompt: Core Label Read
  Out1 : Outport  VectorParamsAs1DForOutWhenUnconnected=off
  wires:
  __CoreLabelRead/1(Out1) -> Out1/1

== system elevator/PLCControllerSuite/__Logic/Task/Program/__Logic/XIO31/Instruction_Enable ==
  Rung-condition-in : Inport  OutDataTypeStr=BOOL
  Enable : EnablePort
  Logical Operator : Logic  OutDataTypeStr=BOOL
  NOT : Logic  DisableCoverage=on  Operator=NOT  IconShape=distinctive  OutDataTypeStr=BOOL
  __CoreVarRead : Subsystem  Tag=CoreVarReadBlock  DisableCoverage=on  TreatAsAtomicUnit=on  mask{PLCBlockType=CoreVarRead}
      mask init:
      | slplc.callbacks.initCoreVariable(gcb, 'read');
      mask Help: web([docroot '/plccoder/ref/__corevarread' '.html']);
      mask DialogControl PLCBlockTitle Prompt: Core Variable Read
  Rung-condition-out : Outport  VectorParamsAs1DForOutWhenUnconnected=off
  wires:
  Rung-condition-in/1 -> Logical Operator/1  "Rung-condition-in"
  Logical Operator/1 -> Rung-condition-out/1  "Rung-condition-out"
  __CoreVarRead/1(y) -> NOT/1  "DataBit"
  NOT/1 -> Logical Operator/2  "~DataBit"

== system elevator/PLCControllerSuite/__Logic/Task/Program/__Logic/XIO31/RungInOverride ==
  In1 : Inport
  AND : Logic  AllPortsSameDT=off  OutDataTypeStr=boolean
  ForceRungInFalseRead : Subsystem  DisableCoverage=on  TreatAsAtomicUnit=on  mask{PLCLabelTag=_Force_RungIn_False, PLCBlockType=ForceRungInFalseRead}
      mask prompts: PLCLabelTag "Label Tag:"
      mask init:
      | block = gcb;
      | maskObj = Simulink.Mask.get(block);
      | maskObj.Display = sprintf('disp(''%s'');', PLCLabelTag);
      mask Help: web([docroot '/plccoder/ref/forcerunginfalseread' '.html']);
      mask DialogControl PLCBlockTitle Prompt: Force Rung-In False Read
      mask Display: disp('_Force_RungIn_False');
  NOT : Logic  Operator=NOT  IconShape=distinctive  AllPortsSameDT=off  OutDataTypeStr=boolean
  Out1 : Outport  VectorParamsAs1DForOutWhenUnconnected=off
  wires:
  AND/1 -> Out1/1
  In1/1 -> AND/2
  ForceRungInFalseRead/1(Out1) -> NOT/1
  NOT/1 -> AND/1

== system elevator/PLCControllerSuite/__Logic/Task/Program/__Logic/XIO31/__CoreVarRead ==
  DataRead : DataStoreRead  DataStoreName=xxx_PLC_VAR_AtFloor3
  y : Outport  VectorParamsAs1DForOutWhenUnconnected=off
  wires:
  DataRead/1 -> y/1

== system elevator/PLCControllerSuite/__Logic/Task/Program/__Logic/XIO32/BlockEnableRead ==
  __CoreLabelRead : Subsystem  Tag=CoreVarReadBlock  DisableCoverage=on  TreatAsAtomicUnit=on  mask{PLCBlockType=CoreLabelRead}
      mask init:
      | slplc.callbacks.initRoutineLabelRead(gcb);
      mask Help: web([docroot '/plccoder/ref/__corelabelread' '.html']);
      mask DialogControl PLCBlockTitle Prompt: Core Label Read
  Out1 : Outport  VectorParamsAs1DForOutWhenUnconnected=off
  wires:
  __CoreLabelRead/1(Out1) -> Out1/1

== system elevator/PLCControllerSuite/__Logic/Task/Program/__Logic/XIO32/Instruction_Enable ==
  Rung-condition-in : Inport  OutDataTypeStr=BOOL
  Enable : EnablePort
  Logical Operator : Logic  OutDataTypeStr=BOOL
  NOT : Logic  DisableCoverage=on  Operator=NOT  IconShape=distinctive  OutDataTypeStr=BOOL
  __CoreVarRead : Subsystem  Tag=CoreVarReadBlock  DisableCoverage=on  TreatAsAtomicUnit=on  mask{PLCBlockType=CoreVarRead}
      mask init:
      | slplc.callbacks.initCoreVariable(gcb, 'read');
      mask Help: web([docroot '/plccoder/ref/__corevarread' '.html']);
      mask DialogControl PLCBlockTitle Prompt: Core Variable Read
  Rung-condition-out : Outport  VectorParamsAs1DForOutWhenUnconnected=off
  wires:
  Rung-condition-in/1 -> Logical Operator/1  "Rung-condition-in"
  Logical Operator/1 -> Rung-condition-out/1  "Rung-condition-out"
  __CoreVarRead/1(y) -> NOT/1  "DataBit"
  NOT/1 -> Logical Operator/2  "~DataBit"

== system elevator/PLCControllerSuite/__Logic/Task/Program/__Logic/XIO32/RungInOverride ==
  In1 : Inport
  AND : Logic  AllPortsSameDT=off  OutDataTypeStr=boolean
  ForceRungInFalseRead : Subsystem  DisableCoverage=on  TreatAsAtomicUnit=on  mask{PLCLabelTag=_Force_RungIn_False, PLCBlockType=ForceRungInFalseRead}
      mask prompts: PLCLabelTag "Label Tag:"
      mask init:
      | block = gcb;
      | maskObj = Simulink.Mask.get(block);
      | maskObj.Display = sprintf('disp(''%s'');', PLCLabelTag);
      mask Help: web([docroot '/plccoder/ref/forcerunginfalseread' '.html']);
      mask DialogControl PLCBlockTitle Prompt: Force Rung-In False Read
      mask Display: disp('_Force_RungIn_False');
  NOT : Logic  Operator=NOT  IconShape=distinctive  AllPortsSameDT=off  OutDataTypeStr=boolean
  Out1 : Outport  VectorParamsAs1DForOutWhenUnconnected=off
  wires:
  AND/1 -> Out1/1
  In1/1 -> AND/2
  ForceRungInFalseRead/1(Out1) -> NOT/1
  NOT/1 -> AND/1

== system elevator/PLCControllerSuite/__Logic/Task/Program/__Logic/XIO32/__CoreVarRead ==
  DataRead : DataStoreRead  DataStoreName=xxx_PLC_VAR_SENCHK
  y : Outport  VectorParamsAs1DForOutWhenUnconnected=off
  wires:
  DataRead/1 -> y/1

== system elevator/PLCControllerSuite/__Logic/Task/Program/__Logic/XIO34/BlockEnableRead ==
  __CoreLabelRead : Subsystem  Tag=CoreVarReadBlock  DisableCoverage=on  TreatAsAtomicUnit=on  mask{PLCBlockType=CoreLabelRead}
      mask init:
      | slplc.callbacks.initRoutineLabelRead(gcb);
      mask Help: web([docroot '/plccoder/ref/__corelabelread' '.html']);
      mask DialogControl PLCBlockTitle Prompt: Core Label Read
  Out1 : Outport  VectorParamsAs1DForOutWhenUnconnected=off
  wires:
  __CoreLabelRead/1(Out1) -> Out1/1

== system elevator/PLCControllerSuite/__Logic/Task/Program/__Logic/XIO34/Instruction_Enable ==
  Rung-condition-in : Inport  OutDataTypeStr=BOOL
  Enable : EnablePort
  Logical Operator : Logic  OutDataTypeStr=BOOL
  NOT : Logic  DisableCoverage=on  Operator=NOT  IconShape=distinctive  OutDataTypeStr=BOOL
  __CoreVarRead : Subsystem  Tag=CoreVarReadBlock  DisableCoverage=on  TreatAsAtomicUnit=on  mask{PLCBlockType=CoreVarRead}
      mask init:
      | slplc.callbacks.initCoreVariable(gcb, 'read');
      mask Help: web([docroot '/plccoder/ref/__corevarread' '.html']);
      mask DialogControl PLCBlockTitle Prompt: Core Variable Read
  Rung-condition-out : Outport  VectorParamsAs1DForOutWhenUnconnected=off
  wires:
  Rung-condition-in/1 -> Logical Operator/1  "Rung-condition-in"
  Logical Operator/1 -> Rung-condition-out/1  "Rung-condition-out"
  __CoreVarRead/1(y) -> NOT/1  "DataBit"
  NOT/1 -> Logical Operator/2  "~DataBit"

== system elevator/PLCControllerSuite/__Logic/Task/Program/__Logic/XIO34/RungInOverride ==
  In1 : Inport
  AND : Logic  AllPortsSameDT=off  OutDataTypeStr=boolean
  ForceRungInFalseRead : Subsystem  DisableCoverage=on  TreatAsAtomicUnit=on  mask{PLCLabelTag=_Force_RungIn_False, PLCBlockType=ForceRungInFalseRead}
      mask prompts: PLCLabelTag "Label Tag:"
      mask init:
      | block = gcb;
      | maskObj = Simulink.Mask.get(block);
      | maskObj.Display = sprintf('disp(''%s'');', PLCLabelTag);
      mask Help: web([docroot '/plccoder/ref/forcerunginfalseread' '.html']);
      mask DialogControl PLCBlockTitle Prompt: Force Rung-In False Read
      mask Display: disp('_Force_RungIn_False');
  NOT : Logic  Operator=NOT  IconShape=distinctive  AllPortsSameDT=off  OutDataTypeStr=boolean
  Out1 : Outport  VectorParamsAs1DForOutWhenUnconnected=off
  wires:
  AND/1 -> Out1/1
  In1/1 -> AND/2
  ForceRungInFalseRead/1(Out1) -> NOT/1
  NOT/1 -> AND/1

== system elevator/PLCControllerSuite/__Logic/Task/Program/__Logic/XIO34/__CoreVarRead ==
  DataRead : DataStoreRead  DataStoreName=xxx_PLC_VAR_AtFloor2
  y : Outport  VectorParamsAs1DForOutWhenUnconnected=off
  wires:
  DataRead/1 -> y/1

== system elevator/PLCControllerSuite/__Logic/Task/Program/__Logic/XIO4/BlockEnableRead ==
  __CoreLabelRead : Subsystem  Tag=CoreVarReadBlock  DisableCoverage=on  TreatAsAtomicUnit=on  mask{PLCBlockType=CoreLabelRead}
      mask init:
      | slplc.callbacks.initRoutineLabelRead(gcb);
      mask Help: web([docroot '/plccoder/ref/__corelabelread' '.html']);
      mask DialogControl PLCBlockTitle Prompt: Core Label Read
  Out1 : Outport  VectorParamsAs1DForOutWhenUnconnected=off
  wires:
  __CoreLabelRead/1(Out1) -> Out1/1

== system elevator/PLCControllerSuite/__Logic/Task/Program/__Logic/XIO4/Instruction_Enable ==
  Rung-condition-in : Inport  OutDataTypeStr=BOOL
  Enable : EnablePort
  Logical Operator : Logic  OutDataTypeStr=BOOL
  NOT : Logic  DisableCoverage=on  Operator=NOT  IconShape=distinctive  OutDataTypeStr=BOOL
  __CoreVarRead : Subsystem  Tag=CoreVarReadBlock  DisableCoverage=on  TreatAsAtomicUnit=on  mask{PLCBlockType=CoreVarRead}
      mask init:
      | slplc.callbacks.initCoreVariable(gcb, 'read');
      mask Help: web([docroot '/plccoder/ref/__corevarread' '.html']);
      mask DialogControl PLCBlockTitle Prompt: Core Variable Read
  Rung-condition-out : Outport  VectorParamsAs1DForOutWhenUnconnected=off
  wires:
  NOT/1 -> Logical Operator/2  "~DataBit"
  __CoreVarRead/1(y) -> NOT/1  "DataBit"
  Logical Operator/1 -> Rung-condition-out/1  "Rung-condition-out"
  Rung-condition-in/1 -> Logical Operator/1  "Rung-condition-in"

== system elevator/PLCControllerSuite/__Logic/Task/Program/__Logic/XIO4/RungInOverride ==
  In1 : Inport
  AND : Logic  AllPortsSameDT=off  OutDataTypeStr=boolean
  ForceRungInFalseRead : Subsystem  DisableCoverage=on  TreatAsAtomicUnit=on  mask{PLCLabelTag=_Force_RungIn_False, PLCBlockType=ForceRungInFalseRead}
      mask prompts: PLCLabelTag "Label Tag:"
      mask init:
      | block = gcb;
      | maskObj = Simulink.Mask.get(block);
      | maskObj.Display = sprintf('disp(''%s'');', PLCLabelTag);
      mask Help: web([docroot '/plccoder/ref/forcerunginfalseread' '.html']);
      mask DialogControl PLCBlockTitle Prompt: Force Rung-In False Read
      mask Display: disp('_Force_RungIn_False');
  NOT : Logic  Operator=NOT  IconShape=distinctive  AllPortsSameDT=off  OutDataTypeStr=boolean
  Out1 : Outport  VectorParamsAs1DForOutWhenUnconnected=off
  wires:
  NOT/1 -> AND/1
  ForceRungInFalseRead/1(Out1) -> NOT/1
  In1/1 -> AND/2
  AND/1 -> Out1/1

== system elevator/PLCControllerSuite/__Logic/Task/Program/__Logic/XIO4/__CoreVarRead ==
  DataRead : DataStoreRead  DataStoreName=xxx_PLC_VAR_AtFloor1
  y : Outport  VectorParamsAs1DForOutWhenUnconnected=off
  wires:
  DataRead/1 -> y/1

== system elevator/PLCControllerSuite/__Logic/Task/Program/__Logic/XIO5/BlockEnableRead ==
  __CoreLabelRead : Subsystem  Tag=CoreVarReadBlock  DisableCoverage=on  TreatAsAtomicUnit=on  mask{PLCBlockType=CoreLabelRead}
      mask init:
      | slplc.callbacks.initRoutineLabelRead(gcb);
      mask Help: web([docroot '/plccoder/ref/__corelabelread' '.html']);
      mask DialogControl PLCBlockTitle Prompt: Core Label Read
  Out1 : Outport  VectorParamsAs1DForOutWhenUnconnected=off
  wires:
  __CoreLabelRead/1(Out1) -> Out1/1

== system elevator/PLCControllerSuite/__Logic/Task/Program/__Logic/XIO5/Instruction_Enable ==
  Rung-condition-in : Inport  OutDataTypeStr=BOOL
  Enable : EnablePort
  Logical Operator : Logic  OutDataTypeStr=BOOL
  NOT : Logic  DisableCoverage=on  Operator=NOT  IconShape=distinctive  OutDataTypeStr=BOOL
  __CoreVarRead : Subsystem  Tag=CoreVarReadBlock  DisableCoverage=on  TreatAsAtomicUnit=on  mask{PLCBlockType=CoreVarRead}
      mask init:
      | slplc.callbacks.initCoreVariable(gcb, 'read');
      mask Help: web([docroot '/plccoder/ref/__corevarread' '.html']);
      mask DialogControl PLCBlockTitle Prompt: Core Variable Read
  Rung-condition-out : Outport  VectorParamsAs1DForOutWhenUnconnected=off
  wires:
  Rung-condition-in/1 -> Logical Operator/1  "Rung-condition-in"
  Logical Operator/1 -> Rung-condition-out/1  "Rung-condition-out"
  __CoreVarRead/1(y) -> NOT/1  "DataBit"
  NOT/1 -> Logical Operator/2  "~DataBit"

== system elevator/PLCControllerSuite/__Logic/Task/Program/__Logic/XIO5/RungInOverride ==
  In1 : Inport
  AND : Logic  AllPortsSameDT=off  OutDataTypeStr=boolean
  ForceRungInFalseRead : Subsystem  DisableCoverage=on  TreatAsAtomicUnit=on  mask{PLCLabelTag=_Force_RungIn_False, PLCBlockType=ForceRungInFalseRead}
      mask prompts: PLCLabelTag "Label Tag:"
      mask init:
      | block = gcb;
      | maskObj = Simulink.Mask.get(block);
      | maskObj.Display = sprintf('disp(''%s'');', PLCLabelTag);
      mask Help: web([docroot '/plccoder/ref/forcerunginfalseread' '.html']);
      mask DialogControl PLCBlockTitle Prompt: Force Rung-In False Read
      mask Display: disp('_Force_RungIn_False');
  NOT : Logic  Operator=NOT  IconShape=distinctive  AllPortsSameDT=off  OutDataTypeStr=boolean
  Out1 : Outport  VectorParamsAs1DForOutWhenUnconnected=off
  wires:
  AND/1 -> Out1/1
  In1/1 -> AND/2
  ForceRungInFalseRead/1(Out1) -> NOT/1
  NOT/1 -> AND/1

== system elevator/PLCControllerSuite/__Logic/Task/Program/__Logic/XIO5/__CoreVarRead ==
  DataRead : DataStoreRead  DataStoreName=xxx_PLC_VAR_AtFloor2
  y : Outport  VectorParamsAs1DForOutWhenUnconnected=off
  wires:
  DataRead/1 -> y/1

== system elevator/PLCControllerSuite/__Logic/Task/Program/__Logic/XIO6/BlockEnableRead ==
  __CoreLabelRead : Subsystem  Tag=CoreVarReadBlock  DisableCoverage=on  TreatAsAtomicUnit=on  mask{PLCBlockType=CoreLabelRead}
      mask init:
      | slplc.callbacks.initRoutineLabelRead(gcb);
      mask Help: web([docroot '/plccoder/ref/__corelabelread' '.html']);
      mask DialogControl PLCBlockTitle Prompt: Core Label Read
  Out1 : Outport  VectorParamsAs1DForOutWhenUnconnected=off
  wires:
  __CoreLabelRead/1(Out1) -> Out1/1

== system elevator/PLCControllerSuite/__Logic/Task/Program/__Logic/XIO6/Instruction_Enable ==
  Rung-condition-in : Inport  OutDataTypeStr=BOOL
  Enable : EnablePort
  Logical Operator : Logic  OutDataTypeStr=BOOL
  NOT : Logic  DisableCoverage=on  Operator=NOT  IconShape=distinctive  OutDataTypeStr=BOOL
  __CoreVarRead : Subsystem  Tag=CoreVarReadBlock  DisableCoverage=on  TreatAsAtomicUnit=on  mask{PLCBlockType=CoreVarRead}
      mask init:
      | slplc.callbacks.initCoreVariable(gcb, 'read');
      mask Help: web([docroot '/plccoder/ref/__corevarread' '.html']);
      mask DialogControl PLCBlockTitle Prompt: Core Variable Read
  Rung-condition-out : Outport  VectorParamsAs1DForOutWhenUnconnected=off
  wires:
  Rung-condition-in/1 -> Logical Operator/1  "Rung-condition-in"
  Logical Operator/1 -> Rung-condition-out/1  "Rung-condition-out"
  __CoreVarRead/1(y) -> NOT/1  "DataBit"
  NOT/1 -> Logical Operator/2  "~DataBit"
